simulink library "lib_trigonometric_function"  (R2023a)
settings: Solver=VariableStepAuto  StartTime=0.0  StopTime=10.0  RelTol=1e-3
libraries: lib_conversion x2
settings Model: Creator=cav2ofo  LastModifiedBy=lenovo
settings OptimizationCC: ReuseModelBlockBuffer=off

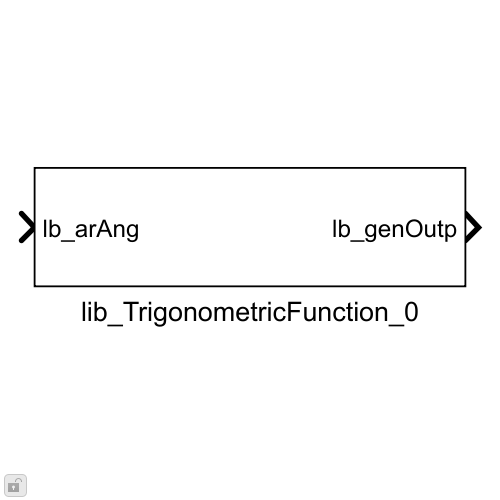
[thumbnail: Simulink's stored preview of the top-level diagram]
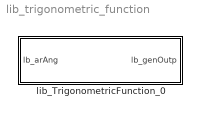
== system lib_trigonometric_function ==
  lib_TrigonometricFunction_0 : Subsystem  mask{lb_parSelSigType=Sine, lb_parLktSizeStr=1024, lb_parOutpDataType=fixdt(1,16,2^-14,0)}
      mask prompts: lb_parSelSigType "Select signal type:"; lb_parLktSizeStr "Lookup data size:"; lb_parOutpDataType "Output data type:"
      mask init:
      | lb_parSinLktSize = str2double(lb_parLktSizeStr);
      | lb_parSinFunLktData = linspace(0,2*pi,lb_parSinLktSize);
      | lb_parSinFunLkt = sin(lb_parSinFunLktData);
      | 
      | Simulink.restoreDiagnostic(gcb);
      | Simulink.suppressDiagnostic([gcb,'/vss_TrigonometricFunctionVariant/vss_CosineFunction/Add'],...
      |             'SimulinkFixedPoint:util:Overflowoccurred');
      | 
      | switch lb_parSelSigType
      |     case 'Sine'
      |         set_param([gcb,'/vss_TrigonometricFunctionVariant'],'LabelModeActiveChoice','lb_parSineFunctLbl');
      |     case 'Cosine'
      |         set_param([gcb,'/vss_TrigonometricFunctionVariant'],'LabelModeActiveChoice','lb_parCosFunctLbl');
      | end
      mask TypeOptions lb_parSelSigType: Sine | Cosine
      mask TypeOptions lb_parLktSizeStr: 128 | 256 | 512 | 1024 | 2048
      mask DialogControl DescGroupVar Prompt: Sine/Cosine block
      mask DialogControl DescTextVar Prompt: VHIT Control Library
      mask DialogControl Control2 Prompt: This block outputs Sine/Cosine performed on the input signal. The input ranges from 0 to 2*pi to output a sensible value.
      mask DialogControl outPar Prompt: Output Parameters

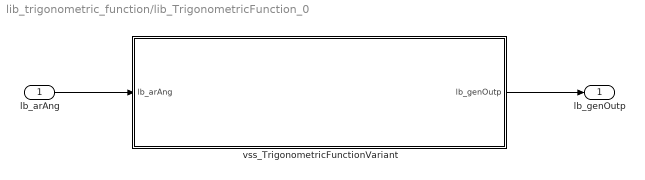
== system lib_trigonometric_function/lib_TrigonometricFunction_0 ==
  lb_arAng : Inport
  vss_TrigonometricFunctionVariant : Subsystem  Variant=on  VariantControlMode=label  LabelModeActiveChoice=lb_parSineFunctLbl
  lb_genOutp : Outport
  wires:
  lb_arAng/1 -> vss_TrigonometricFunctionVariant/1(lb_arAng)
  vss_TrigonometricFunctionVariant/1(lb_genOutp) -> lb_genOutp/1

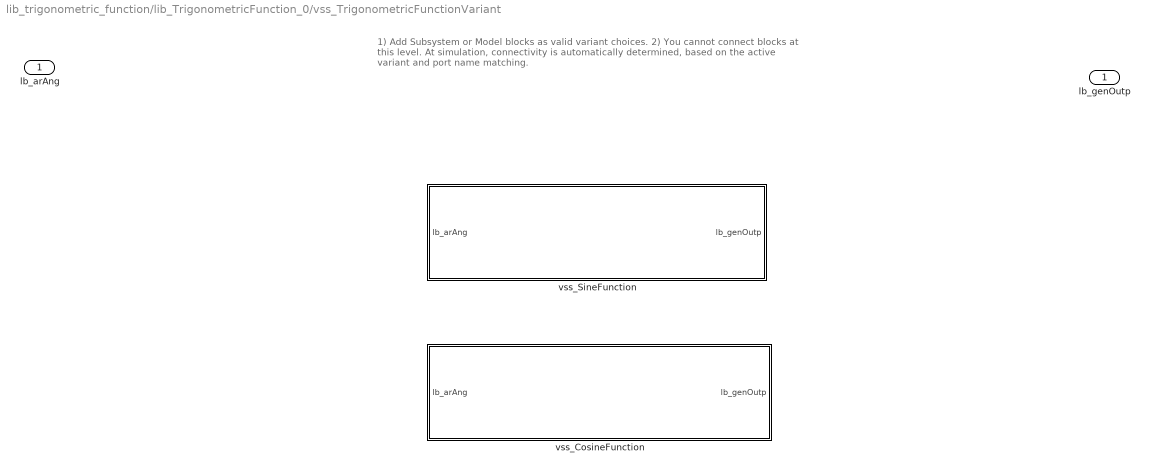
== system lib_trigonometric_function/lib_TrigonometricFunction_0/vss_TrigonometricFunctionVariant ==
  note: 1) Add Subsystem or Model blocks as valid variant choices.
      | 2) You cannot connect blocks at this level. At simulation, connectivity is automatically
      | determined, based on the active variant and port name matching.
  lb_arAng : Inport
  vss_CosineFunction : Subsystem  VariantControl=lb_parCosFunctLbl
  vss_SineFunction : Subsystem  VariantControl=lb_parSineFunctLbl
  lb_genOutp : Outport

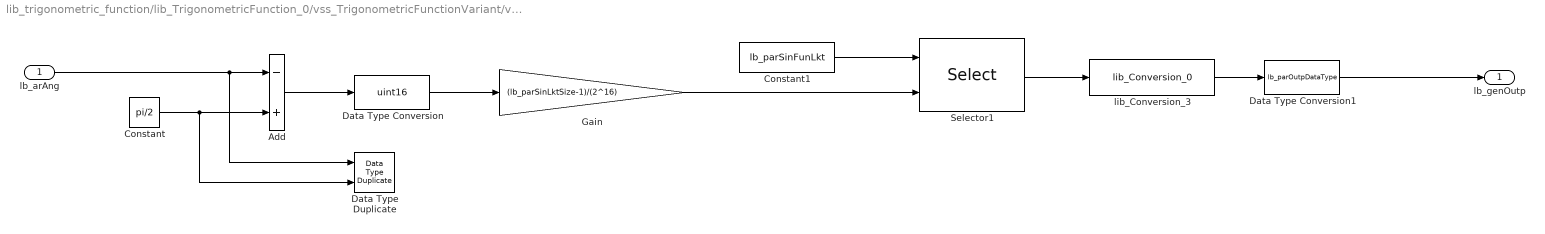
== system lib_trigonometric_function/lib_TrigonometricFunction_0/vss_TrigonometricFunctionVariant/vss_CosineFunction ==
  lb_arAng : Inport
  Add : Sum  Inputs=-+  RndMeth=Simplest  OutDataTypeStr=Inherit: Same as first input
  Constant : Constant  Value=pi/2  OutDataTypeStr=Inherit: Inherit via back propagation
  Constant1 : Constant  Value=lb_parSinFunLkt  OutDataTypeStr=fixdt(1,16,2^-14,0)
  Data Type Duplicate : DataTypeDuplicate
  Data Type Conversion : DataTypeConversion  OutDataTypeStr=uint16  ConvertRealWorld=Stored Integer (SI)  RndMeth=Simplest  SaturateOnIntegerOverflow=off
  Data Type Conversion1 : DataTypeConversion  OutDataTypeStr=lb_parOutpDataType  SaturateOnIntegerOverflow=off  RndMeth=Floor
  Gain : Gain  Gain=(lb_parSinLktSize-1)/(2^16)  OutDataTypeStr=uint16  RndMeth=Simplest
  Selector1 : Selector  IndexMode=Zero-based  InputPortWidth=lb_parSinLktSize  IndexOptions=Index vector (port)  Indices=[1 3]  OutputSizes=1
  lib_Conversion_3 : lib_conversion/lib_Conversion_0  lb_parDataType=fixdt(1,16,2^-14,0)  lb_parOutpMaxVal=[]  lb_parOutpMinVal=[]  lb_parSatFlag=off
      settings: LibrarySourceBlock=vhit_control_library/lib_Conversion_0
  lb_genOutp : Outport
  wires:
  Constant/1 -> Data Type Duplicate/2, Add/2
  Gain/1 -> Selector1/2
  Add/1 -> Data Type Conversion/1
  lb_arAng/1 -> Data Type Duplicate/1, Add/1
  lib_Conversion_3/1 -> Data Type Conversion1/1
  Selector1/1 -> lib_Conversion_3/1
  Data Type Conversion/1 -> Gain/1
  Constant1/1 -> Selector1/1
  Data Type Conversion1/1 -> lb_genOutp/1

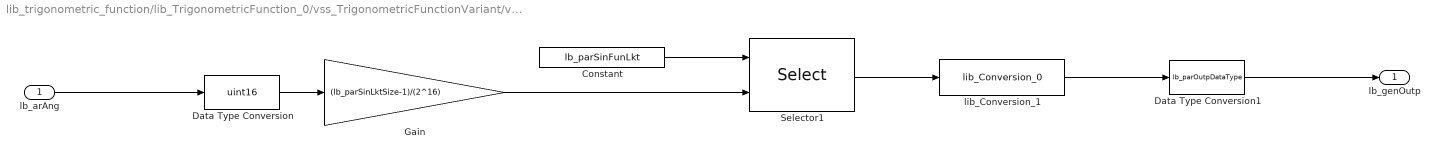
== system lib_trigonometric_function/lib_TrigonometricFunction_0/vss_TrigonometricFunctionVariant/vss_SineFunction ==
  lb_arAng : Inport
  Constant : Constant  Value=lb_parSinFunLkt  OutDataTypeStr=fixdt(1,16,2^-14,0)
  Data Type Conversion : DataTypeConversion  OutDataTypeStr=uint16  ConvertRealWorld=Stored Integer (SI)  RndMeth=Simplest  SaturateOnIntegerOverflow=off
  Data Type Conversion1 : DataTypeConversion  OutDataTypeStr=lb_parOutpDataType  SaturateOnIntegerOverflow=off  RndMeth=Floor
  Gain : Gain  Gain=(lb_parSinLktSize-1)/(2^16)  OutDataTypeStr=uint16  RndMeth=Simplest
  Selector1 : Selector  IndexMode=Zero-based  InputPortWidth=lb_parSinLktSize  IndexOptions=Index vector (port)  Indices=[1 3]  OutputSizes=1
  lib_Conversion_1 : lib_conversion/lib_Conversion_0  lb_parDataType=fixdt(1,16,2^-14,0)  lb_parOutpMaxVal=[]  lb_parOutpMinVal=[]  lb_parSatFlag=off
      settings: LibrarySourceBlock=vhit_control_library/lib_Conversion_0
  lb_genOutp : Outport
  wires:
  lb_arAng/1 -> Data Type Conversion/1
  Data Type Conversion/1 -> Gain/1
  lib_Conversion_1/1 -> Data Type Conversion1/1
  Constant/1 -> Selector1/1
  Selector1/1 -> lib_Conversion_1/1
  Gain/1 -> Selector1/2
  Data Type Conversion1/1 -> lb_genOutp/1
